simulink model "resistenciaBacterias_entrada"  (R2018a)
settings: Solver=VariableStepAuto  StartTime=0.0  StopTime=800  MaxStep=0.05  RelTol=1e-3
libraries: simulink x2
settings Model: Creator=posoriol1  LastModifiedBy=posoriol1
settings CodeAppCC: StateflowObjectComments=on

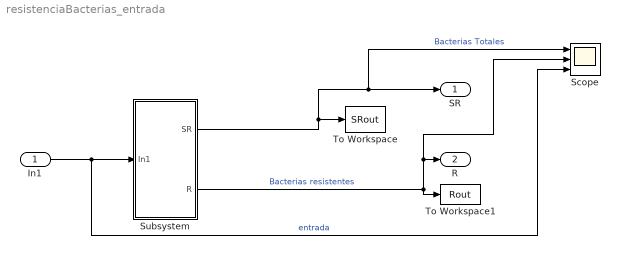
== system resistenciaBacterias_entrada ==
  In1 : Inport
  Scope : Scope  NumInputPorts=3
  Subsystem : Subsystem  mask{par=[0.4,0.1,0.3960,4^(-3),0.2,0.09,0.0083], x0=[0.1,0]}
      mask prompts: par "[bs br alphas q ms mr mc]"; x0 "Cond iniciales (s0,r0)"
      mask init:
      | bs=par(1);br=par(2);alphas=par(3);q=par(4);ms=par(5);mr=par(6);mc=par(7);
  To Workspace : ToWorkspace  VariableName=SRout  SampleTime=-1
  To Workspace1 : ToWorkspace  VariableName=Rout  SampleTime=-1
  SR : Outport
  R : Outport  Port=2
  wires:
  In1/1 -> Scope/3, Subsystem/1(In1)  "entrada"
  Subsystem/1(SR) -> To Workspace/1, Scope/1, SR/1  "Bacterias Totales"
  Subsystem/2(R) -> Scope/2, R/1, To Workspace1/1  "Bacterias resistentes"

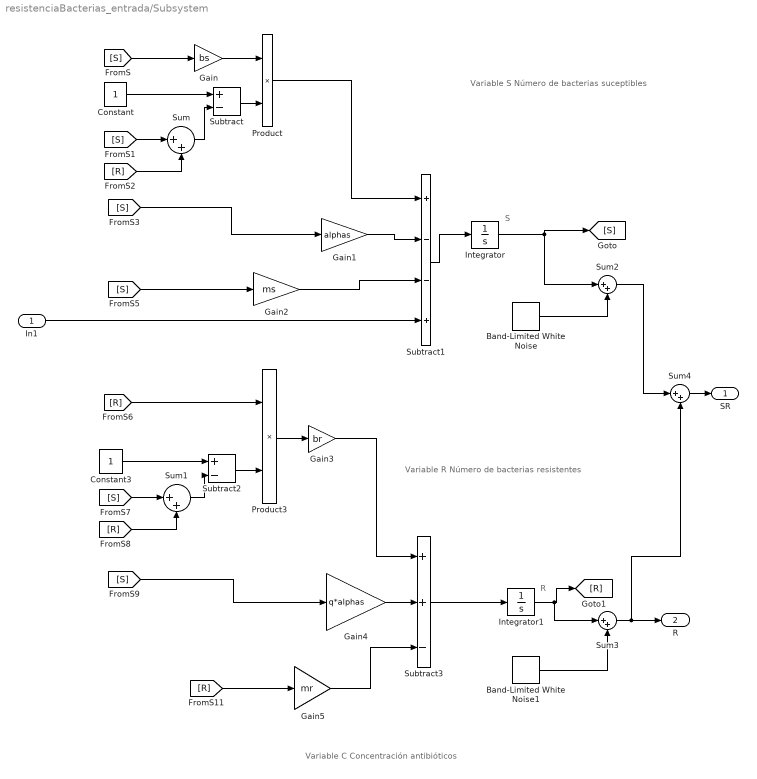
== system resistenciaBacterias_entrada/Subsystem ==
  note: Variable C
      | Concentración antibióticos
  note: R
  note: S
  note: Variable S
      | Número de bacterias suceptibles
  note: Variable R
      | Número de bacterias resistentes
  In1 : Inport
  Band-Limited White Noise : simulink/Sources/Band-Limited White Noise  Cov=[0.000001]  Ts=0.3  seed=[23341]
  Band-Limited White Noise1 : simulink/Sources/Band-Limited White Noise  Cov=[0.0000005]  Ts=0.3  seed=[11558]
  Constant : Constant
  Constant3 : Constant
  Gain : Gain  Gain=bs
  Gain1 : Gain  Gain=alphas
  Gain2 : Gain  Gain=ms
  Gain3 : Gain  Gain=br
  Gain4 : Gain  Gain=q*alphas
  Gain5 : Gain  Gain=mr
  Integrator : Integrator  InitialCondition=x0(1)
  Integrator1 : Integrator  InitialCondition=x0(2)
  Product : Product
  Product3 : Product
  Subtract : Sum  Inputs=+-
  Subtract1 : Sum  Inputs=+--+
  Subtract2 : Sum  Inputs=+-
  Subtract3 : Sum  Inputs=++-
  Sum{,1..4} (5 alike) : Sum  Inputs=|++
  SR : Outport
  R : Outport  Port=2
  wires:
  [S] -> Sum/1
  [R] -> Sum/2
  Constant/1 -> Subtract/1
  [S] -> Sum1/1
  Sum1/1 -> Subtract2/2
  Subtract1/1 -> Integrator/1
  Integrator/1 -> [S], Sum2/1
  [R] -> Sum1/2
  Constant3/1 -> Subtract2/1
  Product3/1 -> Gain3/1
  Product/1 -> Subtract1/1
  Integrator1/1 -> Sum3/1, [R]
  Subtract3/1 -> Integrator1/1
  Sum/1 -> Subtract/2
  [S] -> Gain/1
  Gain/1 -> Product/1
  Subtract/1 -> Product/2
  [S] -> Gain1/1
  Gain1/1 -> Subtract1/2
  [S] -> Gain2/1
  Gain2/1 -> Subtract1/3
  Gain3/1 -> Subtract3/1
  [R] -> Product3/1
  Subtract2/1 -> Product3/2
  Gain4/1 -> Subtract3/2
  [S] -> Gain4/1
  Gain5/1 -> Subtract3/3
  [R] -> Gain5/1
  In1/1 -> Subtract1/4
  Band-Limited White Noise/1 -> Sum2/2
  Band-Limited White Noise1/1 -> Sum3/2
  Sum3/1 -> Sum4/2, R/1
  Sum4/1 -> SR/1
  Sum2/1 -> Sum4/1
